simulink model "float_fmu"  (R2024b)
settings: Solver=ode4  StartTime=0  StopTime=400  FixedStep=0.1  MaxStep=0.1  RelTol=1e-3  EnableMultiTasking=on
undefined symbols (not defined in the file or in its folder): body, pto
libraries: WECSim_Lib_Body_Elements x1, WECSim_Lib_Frames x1, WECSim_Lib_PTOs x1
settings Model: Creator=mlawson  LastModifiedBy=thogan1
settings SolverCC: ZeroCrossControl=DisableAll  AlgebraicLoopSolver=LineSearch  AutoInsertRateTranBlk=on
settings DataIOCC: SaveFormat=Array  SaveOutput=off  SaveTime=off  ReturnWorkspaceOutputs=off
settings OptimizationCC: LifeSpan=inf  SimCompilerOptimization=on
settings DebuggingCC: MergeDetectMultiDrivingBlocksExec=none  SolverPrmCheckMsg=warning  UnconnectedInputMsg=warning  UnconnectedOutputMsg=warning  UnconnectedLineMsg=warning  AllowSymbolicDim=off  StateNameClashWarn=warning  SFUnexpectedBacktrackingDiag=warning  SFNoUnconditionalDefaultTransitionDiag=warning  ArithmeticOperatorsInVariantConditions=warning
settings HardwareCC: ProdBitPerPointer=32  ProdBitPerSizeT=32  ProdBitPerPtrDiffT=32  ProdLargestAtomicFloat=None  ProdIntDivRoundTo=Undefined  ProdEndianess=Unspecified  ProdWordSize=32  ProdHWDeviceType=32-bit Generic
settings ModelReferenceCC: EnableRefExpFcnMdlSchedulingChecks=on  PropagateSignalLabelsOutOfModel=off
settings SFSimCC: SimUseLocalCustomCode=off  CustomCodeUndefinedFunction=UseInterfaceOnly
settings RTWCC: RTWUseLocalCustomCode=off  GPUComputeCapability=3.5  DLArmComputeVersion=19.05
settings CodeAppCC: StateflowObjectComments=on
settings GRTTargetCC: TargetLangStandard=C89/C90 (ANSI)
settings ConfigComp: CovMetricSettings=dw  CovSaveCumulativeToWorkspaceVar=on  CovSaveSingleToWorkspaceVar=on  CovExternalEMLEnable=off  CovSFcnEnable=off
settings SimscapeCC: SimscapeNormalizeSystem=off
settings ConfigurationSet: Description=SimMechanics 2G
settings ExplorerConfigSet: SimMechanicsOpenEditorOnUpdate=off  InternalSimMechanicsExplorerSettings="<ExplorerConfiguration><canonicalview>default</canonicalview><TilePanel><TileInfo><Tiles Columns=\"1\" Count=\"1\" Rows=\"1\"><Column Left=\"2\" Weight=\"1\"/><Column Left=\"1335\"/><Row Top=\"2\" Weight=\"1\"/><Row Top=\"911\"/><Tile Height=\"1\" Width=\"1\" X=\"0\" Y=\"0\"/></Tiles></TileInfo><SceneInfo><SceneViewer><BGColor><R>0.60000002384185791</R><G>0.60000002384185791</G><B>0.60000002384185791</B></BGColor><Camera><Position><X>365.37645888990272</X><Y>-369.82486814446582</Y><Z>359.64809521743916</Z></Position><Center><X>-6.7351450971904585</X><Y>2.2867358426280204</Y><Z>-12.463508769654169</Z></Center><Up><X>-0.40824829046386307</X><Y>0.40824829046386307</Y><Z>0.81649658092772615</Z></Up><Left>-57.820127362122818</Left><Right>57.820127362122818</Right><Bottom>-38.308817187253304</Bottom><Top>38.308817187253304</Top></Camera></SceneViewer></SceneInfo></TilePanel></ExplorerConfiguration>"

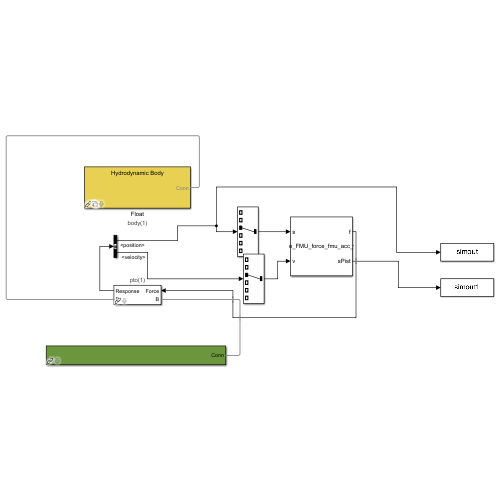
[thumbnail: Simulink's stored preview of the top-level diagram]
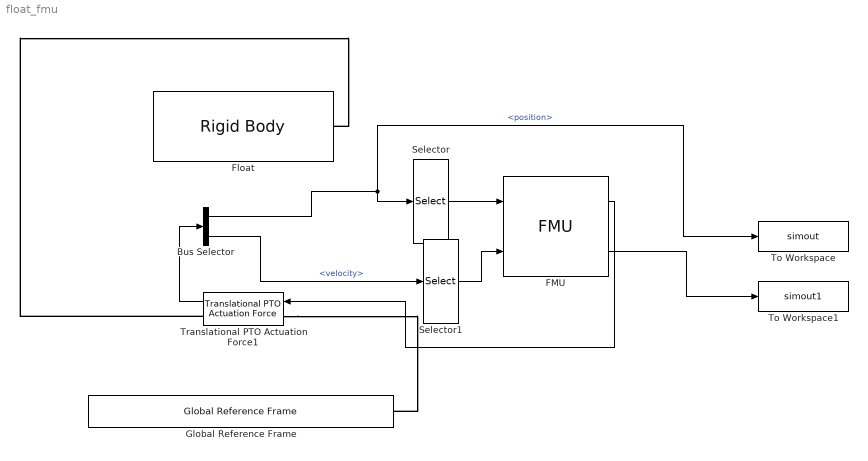
== system float_fmu ==
  Bus Selector : BusSelector  OutputSignals=position,velocity
  FMU : FMU  FMUName=simple_FMU_force_fmu_acc_valve.fmu  FMUMode=ModelExchange  FMUInitializeEnumObject=off  doubleActingCylinder=struct('CHeadExLeakage',2e-9,'CInLeakage',5e-10,'CRodExLeakage',2e-9,'Cst',5.0,'Cv',1000.0,'a_init',0.0,'boreDiameter',0.1484,'closedLength',0.001,'cylinderChamberHead',struct('residualVolume',3e-4,'accumulatorEnable',boolean(false)),'cylinderChamberRod',struct('residualVolume',3e-4,'accumulatorEnable',boolean(false)),'damper',struct('s_nominal',1e-4),'damping',0.0,'dp_nom',1e4,'endOfTravelDistance',0.01,'f_c',200.0,'f_st',2000.0,'maxPressure',2e8,'p_init',1.5e6,'piston',struct('L',0.0),'pistonRodMass',5.0,'q_nom',0.01,'rodDiameter',0.01,'s_init',0.0,'stopDamping',1e12,'stopStiffness',1e9,'stribeckFriction',struct('s_nominal',1e-4,'v_small',0.001),'strokeLength',3.0,'v_init',0.0)  environment=struct('T_ambient',288.15,'p_ambient',101325.0)  fixed=struct('s0',-0.72)  hpAccumulator=struct('Lnom',1.0,'V_init_2',0.5,'damper',struct('s_nominal',1e-4),'fixedLeft',struct('s0',0.0),'gamma',1.4,'gasChamber',struct('stopStiffness',1e9),'gasVolume',1.0,'liquidVolume',0.95,'p_init',7e6,'p_max',2e8,'p_precharge',3e6,'pistonDamping',1.0,'pistonMass',0.01,'liquidChamber',struct('accumulatorEnable',boolean(true)))  laminarRestriction1=struct('L',2.0,'Re_laminar',2000.0,'p_init',3e6)  lpAccumulator=struct('Lnom',1.0,'V_init_2',0.1,'damper',struct('s_nominal',1e-4),'fixedLeft',struct('s0',0.0),'gamma',1.4,'gasChamber',struct('stopStiffness',1e9),'gasVolume',5.0,'liquidVolume',0.48,'p_init',2e5,'p_max',5e7,'p_precharge',1e6,'pistonDamping',1.0,'pistonMass',0.01,'liquidChamber',struct('accumulatorEnable',boolean(true)))  rod=struct('L',2.0)  system=struct('T_ambient',293.15,'dp_small',1.0,'eps_m_flow',1e-4,'m_flow_small',0.01,'m_flow_start',0.0,'p_ambient',101325.0)  v4_3cc=struct('Av',0.001,'Cd',1.0,'Cv',0.0,'Kv',0.0,'bandwidth',10.0,'dampingCoeff',1.0,'p_crack',35000.0,'p_init',3e6,'p_open',4e4,'filterEnable',boolean(true))  mask(simple_FMU_force_fmu_acc_valve [Model Exchange, v2.0]){}
      settings: MultithreadedSim=off
      mask Display:
      | disp('simple_FMU_force_fmu_acc_valve');
      | port_label('output',1,'f');
      | port_label('output',2,'sPist');
      | port_label('input',1,'s');
      | port_label('input',2,'v');
  Float : WECSim_Lib_Body_Elements/Rigid Body  body=body(1)
  Global Reference Frame : WECSim_Lib_Frames/Global Reference Frame  waves=waves  simu=simu
  Selector : Selector  InputPortWidth=6  IndexOptions=Index vector (dialog)  Indices=3  OutputSizes=1
  Selector1 : Selector  InputPortWidth=6  IndexOptions=Index vector (dialog)  Indices=3  OutputSizes=1
  To Workspace : ToWorkspace  VariableName=simout  SaveFormat=Timeseries  SampleTime=-1
  To Workspace1 : ToWorkspace  VariableName=simout1  SaveFormat=Timeseries  SampleTime=-1
  Translational PTO Actuation Force1 : WECSim_Lib_PTOs/Translational PTO Actuation Force  pto=pto(1)
      settings: AttributesFormatString=%<pto>
  wires:
  Translational PTO Actuation Force1/1 -> Bus Selector/1
  Bus Selector/1 -> To Workspace/1, Selector/1  "<position>"
  Bus Selector/2 -> Selector1/1  "<velocity>"
  FMU/1 -> Translational PTO Actuation Force1/1
  Selector/1 -> FMU/1
  Selector1/1 -> FMU/2
  FMU/2 -> To Workspace1/1
  connections:
  Translational PTO Actuation Force1/RConn1 -- Float/RConn1
  Translational PTO Actuation Force1/LConn1 -- Global Reference Frame/RConn1
